simulink model "El_mapa_Logistico"  (R2022b)
settings: Solver=FixedStepAuto  StartTime=0.0  StopTime=1000  FixedStep=1  RelTol=1e-3
settings Model: Creator=scpmoxxa  LastModifiedBy=jibmo
settings DataIOCC: TimeSaveName=t
settings DebuggingCC: UnconnectedInputMsg=warning  UnconnectedOutputMsg=warning  UnconnectedLineMsg=warning
settings ModelReferenceCC: EnableRefExpFcnMdlSchedulingChecks=on
settings RTWCC: DLArmComputeVersion=19.05

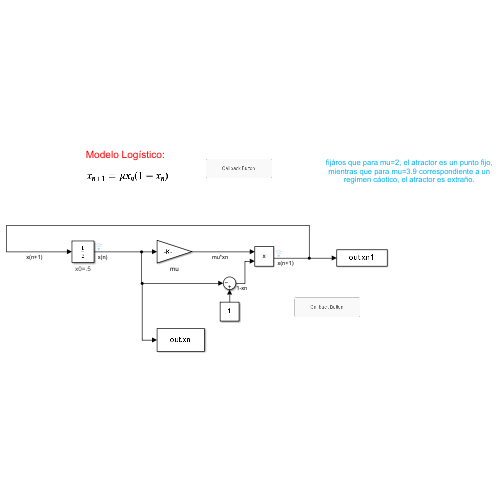
[thumbnail: Simulink's stored preview of the top-level diagram]
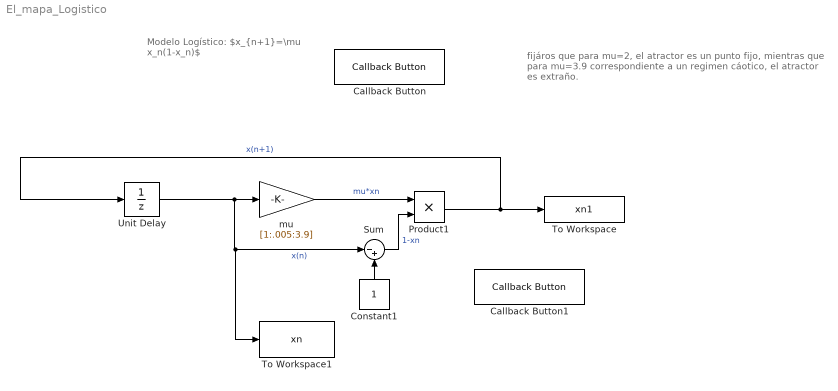
== system El_mapa_Logistico ==
  note: fijáros que para mu=2, el atractor es un punto fijo,
      | mientras que para mu=3.9 correspondiente a un regimen cáotico, el atractor es extraño.
  note: Modelo Logístico:
      |
      | $x_{n+1}=\mu x_n(1-x_n)$
  Callback Button : CallbackButton
      settings: ClickFcn=|
      | close all
      | 
      | figure;
      | plot(out.xn(:,end),out.xn1(:,end),'.','MarkerSize',2,'LineWidth',2)
      | ylabel('$x_{n+1}$','Interpreter','Latex')
      | xlabel('$x_{n}$','Interpreter','Latex')
      | 
      | 
      | 
      | mu=[1:.005:3.9]; %edges of mu pixels
      | 
      | %%%%% bin data and plot image %%%%%%%%%%%%%%%%%%%%%%%%%%%%%%%%%%%%%%%%%%%%%
      | n_x=numel(out.xn(:,1));
      | n_mu=numel(out.xn(1,:));
      | x_data = out.xn;
      | x_edges=linspace(0,1,n_x);     %edges of x pixels
      | 
      | x_histogram=zeros(n_x-1,n_mu-1); %binned values of x
      | for i=1:n_mu-1
      |     x_histogram(:,i)=histcounts(x_data(:,i),x_edges);
      |     x_histogram(:,i)=512*x_histogram(:,i)/max(x_histogram(:,i));
      | end
      | figure1 = figure('InvertHardcopy','off',...
      |     'Colormap',[0.000833433003010255 7.69554144192101e-05 0.125518137504039;0.000871978963804681 8.49428440795541e-05 0.13785734620781;0.000908246049347337 9.50855926993884e-05 0.150487919927737;0.000945709948181513 0.000107171518400248 0.163439930445702;0.000982435954385127 0.000121558697173319 0.176768218976031;0.00102029418433353 0.000137451108883874 0.190686420617748;0.001057227821024 0.000155861710616504 0.20532689255444;0.00109522336612557 0.000175203863194201 0.22085311596022;0.00113430355562725 0.000196420319718818 0.237462932818125;0.0011744914477524 0.00021905271940269 0.255225041939801;0.00121348485126094 0.000243082150504927 0.274034476153509;0.00125350711802938 0.000269175550798264 0.293936883312656;0.00129457847542653 0.000298218480493496 0.31497921879046;0.00133421055716129 0.00032889733386571 0.33658157901379;0.00137224148781413 0.00036382017816364 0.359132824892968;0.00141113475674414 0.000402608914480002 0.381950003215069;0.00144555105949057 0.000446723196683631 0.404941140667108;0.00148063561656653 0.000496893333534474 0.428011003725811;0.00151362286056904 0.000552710673517601 0.451061706264601;0.001544375182624 0.000616132666367999 0.473718238555607;0.00156990618049389 0.000686719856392999 0.496133540805653;0.00159577372213853 0.000766847110946223 0.517910877886086;0.00161905230349668 0.000856041516600218 0.539835356263424;0.00164260175947382 0.000955266357453513 0.560920150398975;0.00166343158796418 0.00106348605819521 0.581685634906705;0.00168447219694855 0.00118357486499408 0.602061400463306;0.00170267597803736 0.00131427500919648 0.621977607337494;0.00171489901453024 0.00145627468500129 0.641365316071875;0.00172719214707424 0.00161320735543758 0.660515555562614;0.00173955567672552 0.0017802269829257 0.67901929513232;0.00174887470365513 0.00196421600341797 0.697560511298916;0.00175510954475535 0.002159424884693 0.715356439215096;0.00176136215525025 0.00236985447008615 0.732733646247066;0.00176449513587962 0.002596377985024 0.750049607565622;0.00176449513587962 0.00283990143247184 0.766882368212333;0.00176136215525025 0.003101364196875 0.783604522219273;0.00175510954475535 0.00337646721437697 0.799780440679256;0.00174887470365513 0.003676391914823 0.8153726976;0.00174265759404831 0.00399123389754927 0.830776028254116;0.00173027641797934 0.00432728582364321 0.845536520469607;0.00171489901453024 0.00468560172521861 0.859619683654479;0.00169355452058195 0.00506726999013671 0.873441085861496;0.00167242308910055 0.00547341391300428 0.886985349471033;0.00164853172355301 0.00590519224617158 0.899777756737098;0.00161905230349668 0.00637255325662883 0.911788173834192;0.00158423527656021 0.00686904779557701 0.922519366631424;0.0015471954433453 0.007396017176253 0.932878300116478;0.00150532147551457 0.00796530740766464 0.941899348438325;0.001461660310351 0.00856912589417599 0.9500298419312;0.00141113475674414 0.009209019989206 0.956767615211995;0.001356926446107 0.0098990342133447 0.962573226895733;0.00129948031939998 0.010629803362243 0.96791976266371;0.00123690146735937 0.0114170640018804 0.973290029606937;0.00116771555364834 0.0122355268510984 0.977701590798467;0.00109094849481932 0.013115865366845 0.982622071999788;0.00101022026857932 0.0140461619353566 0.987067424468369;0.000924954951911635 0.0150285133080348 0.991528850911746;0.000836879784916745 0.0160834341825568 0.99550809271328;0.000746148557320228 0.0171967803268168 0.998001599360128;0.000659173481484325 0.0183913850828432 0.997502498750313;0.000576650390624999 0.0196946361135305 0.992522466275305;0.000502607318204899 0.021047953604832 0.984102072843953;0.000436373247942983 0.0224986804169625 0.974268997572006;0.000376401708396925 0.0240030054235513 0.963543562731098;0.000324828886529677 0.0255601226350274 0.953875333124058;0.000281950621875 0.0271411412588718 0.944762552369437;0.000249570897854697 0.0287994446243124 0.935245529664203;0.000228058627797203 0.0304765235350586 0.924395931036552;0.00021494852891674 0.032198817702743 0.912717337288918;0.000205798270887181 0.0339646942486052 0.900697116787804;0.000198595495834735 0.035807211348974 0.888348963053934;0.000192127145300718 0.0376925174352893 0.875686896373931;0.000186346939556218 0.0396564117424901 0.862725242858644;0.000181213731048656 0.0416619777034918 0.848601324443055;0.000177688279879503 0.043788794519238 0.83293366273506;0.000175203863194201 0.0459590334293163 0.816222398128136;0.000172747314004295 0.0481702872164663 0.798526735563776;0.000170801981216778 0.0505117163936704 0.78031897329754;0.000166489022710968 0.052848099871532 0.762847428375716;0.000159494694624 0.055319479432175 0.746481347592814;0.000148794342125046 0.0578313121592078 0.73117546787198;0.000136234735043982 0.0604335691138031 0.717270793823114;0.000121927951752832 0.0631286700228359 0.704333623262873;0.000108175616801 0.0659190774006813 0.691583804459687;9.63038419237908e-05 0.0687485575585739 0.678652535232093;8.66170930239999e-05 0.0716136856894527 0.665554338741556;7.92856589707878e-05 0.0745735518718749 0.652659166737422;7.39339851068722e-05 0.0775657943028243 0.640314586749711;6.98168260742186e-05 0.0805866256523103 0.628502271121256;6.65657883308329e-05 0.0837008503669129 0.617204725664768;6.32181037375497e-05 0.0869106174435908 0.607075765315625;5.95883203587814e-05 0.090145152017568 0.597742469954267;5.53367022390476e-05 0.0935503855567254 0.589834191535207;5.05953844842714e-05 0.0970577565107565 0.582334186113183;4.55085839062901e-05 0.10058990186932 0.575231847327263;4.02266704911059e-05 0.10430607807795 0.56851715230788;3.54469861133516e-05 0.108046950860063 0.561550114565451;3.08855510988149e-05 0.111894393218928 0.554339595821369;2.69164963400209e-05 0.115761550173451 0.546586282919581;2.33663970299062e-05 0.119734897198256 0.538005821041818;2.02890819089203e-05 0.12372262079704 0.528932398370928;1.7544881231416e-05 0.127815891333067 0.518797610148157;1.50365669017812e-05 0.131917856846594 0.508236601090536;1.26417271688397e-05 0.136023078872351 0.496990321986647;1.04581732286405e-05 0.140126044921875 0.485102506461781;8.32501777613822e-06 0.144221179597632 0.472893711768106;6.37868239809822e-06 0.148411502624003 0.460125304108904;4.56909905784374e-06 0.152476427466815 0.447108747722967;3.05763060002948e-06 0.156629937551694 0.43387547783519;1.84267035634793e-06 0.160757586555356 0.42045716956898;9.76783283783677e-07 0.164735383850157 0.407129218102417;4.38297415843749e-07 0.168791535858854 0.393666829866811;1.5220870177393e-07 0.172804411773707 0.380332160920014;3.79637599436799e-08 0.176768218976031 0.366912709774417;7.01583371423998e-09 0.180804432571036 0.353874748455313;8.94660968749997e-10 0.18465502055271 0.340998599643224;6.24032145099998e-11 0.188570935580053 0.328294860972832;2.05962975999999e-12 0.192419195094466 0.315773717614195;2.47609899999999e-14 0.196194120249632 0.303444927715911;5.90489999999996e-16 0.200028060201706 0.291504263973251;1.88956799999999e-14 0.203781609614355 0.279942489366806;2.05962975999999e-12 0.207449189412029 0.268575797077869;7.33904022399997e-11 0.211169386259126 0.257412480053396;1.11577100832e-09 0.214796644129374 0.24662348925525;1.036579476493e-08 0.218325538604853 0.236041759621536;6.84119281284898e-08 0.2219006624 0.225826406837776;3.25201606410239e-07 0.225370621719697 0.215821156107377;1.05706913843168e-06 0.228883854949054 0.206173716641847;2.70678415699999e-06 0.23228520357288 0.196738196787935;5.87216781904498e-06 0.235569550331114 0.187651335446609;1.12041307564134e-05 0.238890943128751 0.178903379454911;1.9338742116417e-05 0.242249694483482 0.170363365954737;3.07625012510003e-05 0.245646118665658 0.162152639684375;4.55085839062901e-05 0.248916122117045 0.154261584969137;6.36565077691596e-05 0.252387010442144 0.146680775178125;8.43905517787442e-05 0.255896509713547 0.139194359099457;0.00010784008474947 0.259444941176763 0.132115783077813;0.000133033121788223 0.263032627854232 0.125138412665244;0.000159953539817247 0.266833614345345 0.118459000371037;0.00018843250287609 0.270502696142371 0.111981119608514;0.000218462599273245 0.274389673093685 0.105624097399537;0.000250885117684406 0.278321205181411 0.0994801738644885;0.00028485431128597 0.282297674353218 0.0934752808836914;0.000322407210808102 0.286319464733387 0.0876925662645397;0.000371868985430063 0.290201079289406 0.0820642540167904;0.000426216029353375 0.293936883312656 0.0766646247382421;0.000490105275284623 0.297900783482813 0.0714318636294193;0.000569002615795721 0.301715572831774 0.0663745538317944;0.000669217298019135 0.305182203293901 0.0615003312645508;0.000797922662976119 0.308680625302872 0.0568662934977131;0.000959110482694533 0.312014078444351 0.05246858187476;0.00116321569174572 0.31497921879046 0.0482587054878407;0.00142165379145934 0.317766980549496 0.044240899506176;0.00174887470365513 0.320373257272842 0.0404952676599386;0.00215574237380985 0.322591900156152 0.036936242722357;0.00264802844774444 0.324619498420242 0.033631970578834;0.00323148741402853 0.326453041818118 0.0304765235350586;0.00391947249978916 0.328089804851206 0.0275624922521815;0.00470618266742554 0.329527351868225 0.0247977383536514;0.00562235230672084 0.330969933440625 0.0221880619437221;0.00666686901440087 0.332003438548233 0.0197811867870156;0.00787152539961871 0.333039523869309 0.017528754699968;0.00926796129684563 0.333662415572717 0.0154685313879058;0.010896201253125 0.334078194232095 0.0135906848655028;0.0128220769612081 0.333870253124243 0.011899807533762;0.0150807802873686 0.333454681538834 0.0104074851209159;0.0177065697361678 0.33262477980639 0.00906878372779393;0.0207760198747344 0.331383026166809 0.00789228910582738;0.024257110773438 0.329939003724258 0.00685046774751219;0.0282187126574992 0.328089804851206 0.00592995538828549;0.0326494138986731 0.32624890660576 0.00510383022796799;0.0375475185019341 0.324010151517171 0.0043724554301111;0.0429762582970356 0.321581907523757 0.00372173693419261;0.048970736047507 0.31896776132125 0.0031459232966592;0.0555171546975816 0.316171567781183 0.002639363440625;0.0627456752360546 0.31339501871623 0.0022002656693549;0.0706482305178633 0.310245741246862 0.00182487395382829;0.0793276914660124 0.306927426743077 0.00150532147551457;0.0887679200628284 0.303444927715911 0.00123926286695281;0.0990075848201625 0.299803324129956 0.00101827299997596;0.110171118099438 0.29600791387914 0.000835154971437282;0.12213357832379 0.292064202847648 0.000685247473023425;0.135113296385789 0.287977894573924 0.000562691646576751;0.148955692061092 0.283754879536546 0.000464768164723468;0.163674859155563 0.279581552734375 0.000384671937792968;0.179282304861539 0.275457474395955 0.000318403196801599;0.195922533746098 0.271206122354814 0.000263648520462346;0.21363054132644 0.267007424666665 0.00021787375163948;0.23228520357288 0.262689243269417 0.000179696036660944;0.251888812787799 0.258427112141436 0.000149228397670483;0.272440639012851 0.254220483851361 0.000125291794955247;0.294124678401921 0.250068814543926 0.000107505385800007;0.316569818855217 0.245971563928238 9.53889925569998e-05;0.340153707591776 0.24192819526606 8.83176384688296e-05;0.364453218457789 0.238096758515859 8.52200724470936e-05;0.389416118118107 0.234314019279471 8.54980241758616e-05;0.415480812253011 0.230579511866205 8.83176384688296e-05;0.442401831284641 0.227198188479256 9.35801514286181e-05;0.4704270176 0.223856650166943 0.000100666422249167;0.499280859972098 0.220703789991403 0.000109865828057594;0.528932398370928 0.217734191339699 0.000122298103125;0.559347713201003 0.21494276429004 0.000139909921428094;0.59049 0.212469508526688 0.000163662449693837;0.621635711123609 0.210306179677595 0.000196962318063843;0.653370279294392 0.208445581378743 0.000241162079949;0.685278513171595 0.207023332454174 0.00029897537980061;0.717270793823114 0.205891132094649 0.000371868985430063;0.749652461748224 0.205186026140596 0.000460470753987357;0.783193224452664 0.205045237051526 0.000560182994103149;0.817923924320878 0.205186026140596 0.000660600881299127;0.85387594607202 0.206173716641847 0.00075246913582143;0.890169722768657 0.207875746888349 0.000826573509448014;0.92345726749599 0.211602051158893 0.000875552643290349;0.9509900499 0.216702417311206 0.000845546651542831;0.973290029606937 0.222952180036757 0.000786358762139441;0.983115207627714 0.230734159420579 0.000718229345527367;0.985583856463435 0.239368470181339 0.000656326084096105;0.986078180787156 0.248423414191436 0.00059876664661656;0.985583856463435 0.257919396950346 0.000544093972190985;0.984595802551474 0.267703571921664 0.000493489967354548;0.983115207627714 0.277782449622624 0.000446723196683631;0.981143852321775 0.288347476012134 0.000403571172440593;0.978684106637931 0.299231544275905 0.000364707544030055;0.97475877686915 0.310638010435879 0.000329715893276088;0.969382024099007 0.322389698896272 0.000299733815178786;0.962088352219452 0.334702639280589 0.000274087383738136;0.953875333124058 0.347603599857628 0.000251544300499197;0.943807378499177 0.360899338082654 0.000231742858886718;0.932405429941632 0.374826842620627 0.000214367273094669;0.920177948127332 0.389181048634368 0.000198049904143088;0.907153700496149 0.403971686621693 0.000182231211538777;0.893820198584142 0.419208633898092 0.000167439842754005;0.880192376136458 0.4351588284463 0.000153180667225774;0.867623536069632 0.451326227548824 0.000139909921428094;0.856081430861085 0.467970627544737 0.000127959103652906;0.845973806621025 0.48538288011425 0.000117197000509942;0.837262380475962 0.503020990287943 0.000107505385800007;0.82991422746916 0.521168168729709 9.90905857871842e-05;0.823473492164723 0.539835356263424 9.15046286419954e-05;0.818775750870958 0.559033649360975 8.43905517787442e-05;0.815797459362816 0.578451540653379 7.77259898552429e-05;0.813675419467899 0.598073812778693 7.10082119679999e-05;0.8132515418883 0.618565405748432 6.40973406249999e-05;0.814099473773607 0.638915756947392 5.73298960392156e-05;0.815797459362816 0.660156813687765 5.04127298574242e-05;0.818775750870958 0.681591056641668 4.38527005714021e-05;0.823045535884519 0.703201132946432 3.77040460326502e-05;0.827762854126324 0.725742705335569 3.18841932604229e-05;0.833365727080329 0.748462033561057 2.65869105666457e-05;0.839868237097985 0.771340503351216 2.17377311870156e-05;0.847286750713731 0.79519120666402 1.73109528309657e-05;0.855198690751778 0.819201930203214 1.3445498838013e-05;0.863614192028781 0.844225746868247 1.005010010005e-05;0.872095812856093 0.869410239615807 7.26129685547166e-06;0.880643942090494 0.895649922021691 5.04176297541631e-06;0.889714253210675 0.922050702057364 3.38048802503124e-06],...
      |     'Color',[1 1 1]);
      | 
      | %olormap(flipud(gray(512)));
      | brighten(0.5);
      | %cmap=colormap;
      | im=image([mu(1) mu(end)], [x_edges(1) x_edges(end)], 5+x_histogram);
      | 
      | set(gca,'YDir','normal');
      | xlabel('$\mu$','Interpreter','latex','FontSize',14);
      | ylabel('$x\;\;$','Interpreter','latex','FontSize',14);
      | title('Diagrama de bifurcación del Mapa Logístico','FontSize',14)
  Callback Button1 : CallbackButton
  Constant1 : Constant
  Product1 : Product
  Sum : Sum  Inputs=|-+
  To Workspace : ToWorkspace  VariableName=xn1  SampleTime=-1
  To Workspace1 : ToWorkspace  VariableName=xn  SampleTime=-1
  Unit Delay : UnitDelay  InitialCondition=.5  SampleTime=-1  HasFrameUpgradeWarning=on
      settings: AttributesFormatString=x0=%<InitialCondition>
  mu : Gain  Gain=[1:.005:3.9]
  wires:
  Product1/1 -> To Workspace/1, Unit Delay/1  "x(n+1)"
  mu/1 -> Product1/1  "mu*xn"
  Sum/1 -> Product1/2  "1-xn"
  Unit Delay/1 -> To Workspace1/1, Sum/1, mu/1  "x(n)"
  Constant1/1 -> Sum/2
